simulink model "motor3"  (R2021a)
settings: Solver=VariableStepAuto  StartTime=0.0  StopTime=10.0  RelTol=1e-3
libraries: nesl_utility x12, ee_lib x10, fl_lib x7, pid_lib x3, eeTransforms x2, embmathops x2, eePwmGeneratorTwoLevel x1
settings Model: Creator=Sujit  LastModifiedBy=Sujit

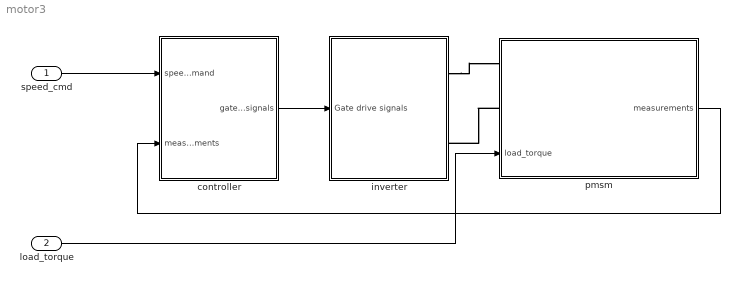
== system motor3 ==
  speed_cmd : Inport
  load_torque : Inport  Port=2
  controller : Subsystem
  inverter : Subsystem
  pmsm : Subsystem
      settings: PortSchema="{\"entries\":[{\"content\":{\"sides\":[{\"content\":{\"connectorIds\":[\"LConn1\",\"LConn2\",\"In1\"]},\"type\":\"ConnectorPlacement.EquallySpacedRectSide\",\"uuid\":\"9aa95156-5b90-445e-ac58-1a81c189d6db\"},{\"content\":{\"connectorIds\":[\"Out1\"],\"side\":\"RIGHT\"},\"type\":\"ConnectorPlacement.EquallySpacedRectSide\",\"uuid\":\"e0f82fa8-5145-4e03-9494-9a86df107329\"},{\"content\":{\"connectorIds\":[],\"side\":\"TOP\"},\"type\":\"ConnectorPlacement.EquallySpacedRectSide\",\"uuid\":\"ed322135-5092-4528-967b-f1137f8969df\"}]},\"type\":\"ConnectorPlacement.EquallySpacedConnector\",\"uuid\":\"a6e6cb3b-bfcb-454a-ab1c-5c06ba05c769\"}],\"packageUris\":[\"http://schema.mathworks.com/mf0/Connector/R2020b\"],\"version\":\"1.0\"}"
  wires:
  load_torque/1 -> pmsm/1(load_torque)
  pmsm/1(measurements) -> controller/2(measurements)
  speed_cmd/1 -> controller/1(speed_command)
  controller/1(gate_signals) -> inverter/1(Gate drive signals)
  connections:
  inverter/RConn1 -- pmsm/LConn1
  pmsm/LConn2 -- inverter/RConn2

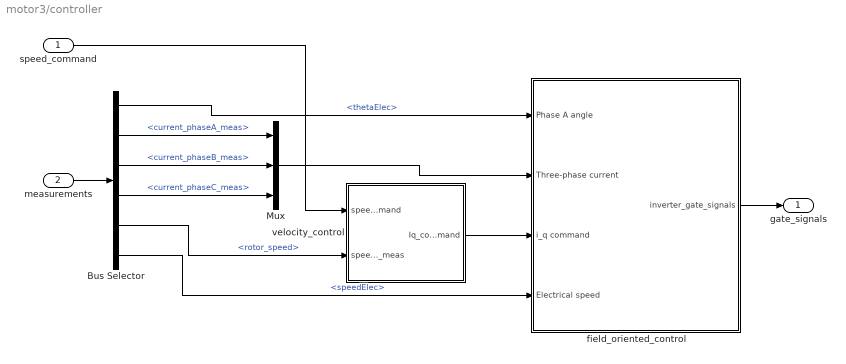
== system motor3/controller ==
  speed_command : Inport
  measurements : Inport  Port=2
  Bus Selector : BusSelector  OutputSignals=thetaElec,current_phaseA_meas,current_phaseB_meas,current_phaseC_meas,rotor_speed,speedElec
  Mux : Mux  Inputs=3
  field_oriented_control : Subsystem
  velocity_control : Subsystem
  gate_signals : Outport
  wires:
  velocity_control/1(Iq_command) -> field_oriented_control/3(i_q command)
  speed_command/1 -> velocity_control/1(speed_command)
  measurements/1 -> Bus Selector/1
  Bus Selector/5 -> velocity_control/2(speed_meas)  "<rotor_speed>"
  Bus Selector/2 -> Mux/1  "<current_phaseA_meas>"
  Bus Selector/3 -> Mux/2  "<current_phaseB_meas>"
  Bus Selector/4 -> Mux/3  "<current_phaseC_meas>"
  Mux/1 -> field_oriented_control/2(Three-phase current)
  field_oriented_control/1(inverter_gate_signals) -> gate_signals/1
  Bus Selector/1 -> field_oriented_control/1(Phase A angle)  "<thetaElec>"
  Bus Selector/6 -> field_oriented_control/4(Electrical speed)  "<speedElec>"

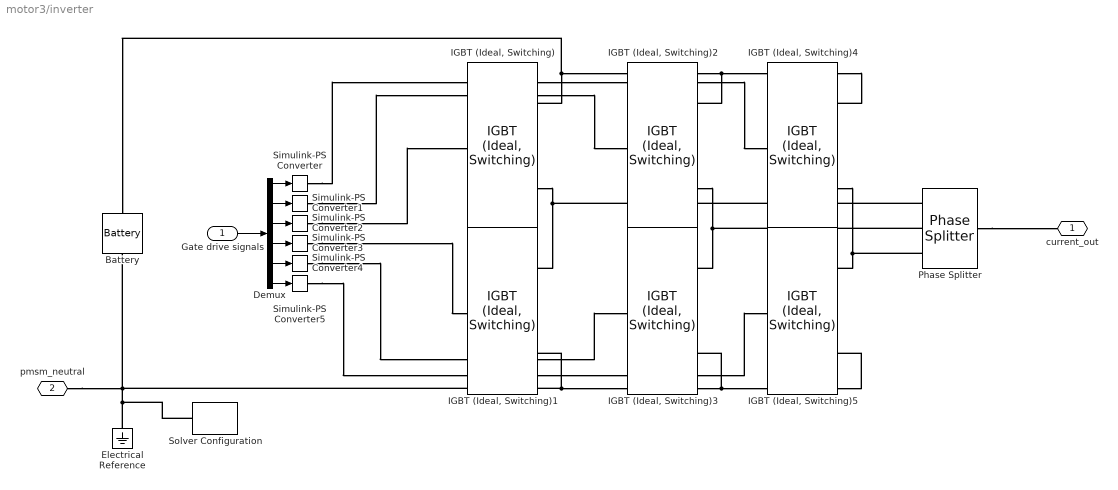
== system motor3/inverter ==
  Gate drive signals : Inport
  Battery : ee_lib/Sources/Battery  Vnom=400 V  prm_dir=1  R1_dis=2 Ohm  R1_ch=2 Ohm  R1=2 Ohm  prm_AH=1  AH=50 hr*A  V1=11.5 V  AH1=25 hr*A  prm_R2=1  R2=2000 Ohm  prm_dyn=1  Rp1=0.005 Ohm  tau1=30 s  Rp2=0.005 Ohm  tau2=30 s  Rp3=0.005 Ohm  tau3=30 s  Rp4=0.005 Ohm  tau4=30 s  Rp5=0.005 Ohm  tau5=30 s  prm_fade=1  N_fade=100  AH_fade=45 hr*A  R1_fade=2.02 Ohm  R1_ch_fade=2.02 Ohm  V1_fade=10.35 V  prm_age=1  prm_age_OCV=1  OCV_age=0.9  SOC_age=60  Tmeas_age=298.15 K  delta_time_age_vec=[0] d  temperature_age_vec=[273] K  OCV_scaling_age=2.2134e6  OCV_offset_age=1.632e6  temp_exp_age=0.515833569 V  t_exp_age=0.75  i_specify=off  i_priority=None  i=0 A  i_nominal_specify=off  i_nominal_unit=A  i_nominal_value=1  v_specify=off  v_priority=None  v=0 V  v_nominal_specify=off  v_nominal_unit=V  v_nominal_value=1  charge_specify=off  charge_priority=High  charge=50 hr*A  charge_nominal_specify=off  charge_nominal_unit=hr*A  charge_nominal_value=1  num_cycles_specify=off  num_cycles_priority=High  num_cycles=0  num_cycles_nominal_specify=off  num_cycles_nominal_unit=1  num_cycles_nominal_value=1  thermal_mass=30000 J/K  Tmeas=298.15 K  Vnom_T2=12 V  R1_T2=2.2 Ohm  R1_T2_dis=2.2 Ohm  R1_T2_ch=2.2 Ohm  V1_T2=11.4 V  R2_T2=2200 Ohm  Rp1_T2=0.005 Ohm  tau1_T2=30 s  Rp2_T2=0.005 Ohm  tau2_T2=30 s  Rp3_T2=0.005 Ohm  tau3_T2=30 s  Rp4_T2=0.005 Ohm  tau4_T2=30 s  Rp5_T2=0.005 Ohm  tau5_T2=30 s  Tmeas2=273.15 K  temperature_specify=off  temperature_priority=High  temperature=298.15 K  temperature_nominal_specify=off  temperature_nominal_unit=K  temperature_nominal_value=1
  Demux : Demux  Outputs=6
  Electrical Reference : fl_lib/Electrical/Electrical Elements/Electrical Reference
  IGBT (Ideal, Switching){,1..5} (6 alike) : ee_lib/Semiconductors & Converters/IGBT (Ideal, Switching)  Vf=0.8 V  Ron=0.021 Ohm  Goff=0.12195 1/Ohm  Vth=5.8 V  diode_param=ee.enum.converters.protectiondiode.chargedynamics  diode_Vf=2.22 V  diode_Ron=0.0184 Ohm  diode_Goff=1 1/Ohm  diode_C=50e-9 F  diode_iRM=-35 A  diode_iF=50 A  diode_idot=-1380 A/us  diode_trr_param=ee.enum.converters.diodetrr.Qrr  diode_trr_factor=3  diode_trr=15 us  diode_Qrr=8.7 uC  thermal_loss_option=ee.enum.converters.thermalLossOption.constantvalues  Von_data=[0, .1, .6, .8, 1, 1.3, 1.6, 2, 2.4; 0, .1, .7, 1, 1.2, 1.5, 1.9, 2.4, 2.8] V  Eon_data=[0, .0024, .024, .12, .2, .48, 1.04, 2.16, 3.24; 0, .003, .03, .15, .25, .6, 1.3, 2.7, 4.05] * 1e-3 J  Eoff_data=[0, .0007, .0066, .033, .066, .17, .33, .83, 1.5; 0, .001, .01, .05, .1, .25, .5, 1.2, 2.2] * 1e-3 J  Tj=[298.15, 398.15] K  Iout_data=[0, .1, 1, 5, 10, 20, 40, 70, 100] A  Eon_scalar=5.5e-3 J  Eoff_scalar=4.5e-3 J  Voff=600 V  Iout_scalar=50 A  diodeModelType=ee.enum.converters.diodeModelType.pwl  diode_IfMat=[.07, .12, .19, 1.75, 4.24, 7.32, 11.2; .16, .3, .72, 2.14, 4.02, 6.35, 9.12] A  diode_TjVec=[25, 125] degC  diode_VfVec=[.5, .7, .9, 1.3, 1.7, 2.1, 2.5] V  thermal_network_parameterization=ee.enum.thermalNetworkTopology.cauer  Rth=[.53, .5] K/W  Rth_Foster=[.08, .14, .22, .16] K/W  thermal_mass_parameterization=ee.enum.thermalNetwork.timeconstant  thermal_mass=[.01, .5] J/K  thermal_mass_Foster=[.001, .005, .05, .5] J/K  thermal_time_constant=[.001, .2] s  thermal_time_constant_Foster=[7e-05, .0007, .01, .08] s  thermal_mass_initial_temperatures=[25, 25] degC  junction_thermal_mass=0.01 J/K  vT_specify=off  vT_priority=None  vT=0 V  vT_nominal_specify=off  vT_nominal_unit=V  vT_nominal_value=1  Qj_specify=off  Qj_priority=None  Qj=0 W  Qj_nominal_specify=off  Qj_nominal_unit=W  Qj_nominal_value=1  junction_temperature_specify=on  junction_temperature_priority=None  junction_temperature=25 degC  junction_temperature_nominal_specify=off  junction_temperature_nominal_unit=degC  junction_temperature_nominal_value=1
  Phase Splitter : ee_lib/Connectors & References/Phase Splitter
      settings: SourceProductBaseCode=PS
  Simulink-PS Converter{,1..5} (6 alike) : nesl_utility/Simulink-PS Converter  PhysicalDomain=network_engine_domain  SubClassName=ps_input  LeftPortType=input  RightPortType=output  PseudoPeriodic=off  Frequencies=[]  NoiseDistribution=none  NoiseParameters=[]  Unit=1  AffineConversion=off  FilteringAndDerivatives=provide  SimscapeFilterOrder=1  InputFilterTimeConstant=0.001  UdotUserProvided=0
      settings: SourceProductBaseCode=PW,SS
  Solver Configuration : nesl_utility/Solver Configuration  PhysicalDomain=network_engine_domain  SubClassName=solver  LeftPortType=input  RightPortType=generic  Tones=[]  Harmonics=[]  SimulateNoise=off  Profile=off  UseLocalSampling=off  EnableSwitchedLinearOptims=on  FrequencyDomain=off  UseCCode=off  RelTol=0.001  AbsTol=1e-06  MinStep=1e-09  ToWorkspace=off  RevertToSquareIcSolve=off  NumHomotopyIterations=100  PhasorMode=off  PhasorModeNumHarmonics=1  DoDC=off  ResidualTolerance=1e-09  UseLocalSolver=off  LocalSolverChoice=NE_BACKWARD_EULER_ADVANCER  LocalSolverSampleTime=0.001  DoFixedCost=off  MaxNonlinIter=3  MaxModeIter=2  ComputeImpulses=off  ImpulseIterations=2  LinearAlgebra=auto  EquationFormulation=NE_TIME_EF  DelaysMemoryBudget=1024  AutomaticFiltering=on  FilteringTimeConstant=0.001  PartitionStorageMethod=AS_NEEDED  PartitionMemoryBudget=1024  PartitionMethod=ROBUST
      settings: SourceProductBaseCode=PW,SS
  current_out : PMIOPort  Side=Right
  pmsm_neutral : PMIOPort  Port=2  Side=Right
  wires:
  Demux/1 -> Simulink-PS Converter/1
  Demux/2 -> Simulink-PS Converter1/1
  Demux/6 -> Simulink-PS Converter5/1
  Demux/3 -> Simulink-PS Converter2/1
  Demux/4 -> Simulink-PS Converter3/1
  Demux/5 -> Simulink-PS Converter4/1
  Gate drive signals/1 -> Demux/1
  connections:
  "IGBT (Ideal, Switching)2"/RConn2 -- Phase Splitter/RConn2 -- "IGBT (Ideal, Switching)3"/RConn1
  Battery/LConn1 -- "IGBT (Ideal, Switching)"/RConn1 -- "IGBT (Ideal, Switching)4"/RConn1 -- "IGBT (Ideal, Switching)2"/RConn1
  Solver Configuration/RConn1 -- Electrical Reference/LConn1 -- pmsm_neutral/RConn1 -- Battery/RConn1 -- "IGBT (Ideal, Switching)1"/RConn2 -- "IGBT (Ideal, Switching)5"/RConn2 -- "IGBT (Ideal, Switching)3"/RConn2
  "IGBT (Ideal, Switching)"/RConn2 -- Phase Splitter/RConn1 -- "IGBT (Ideal, Switching)1"/RConn1
  "IGBT (Ideal, Switching)4"/RConn2 -- Phase Splitter/RConn3 -- "IGBT (Ideal, Switching)5"/RConn1
  Simulink-PS Converter/RConn1 -- "IGBT (Ideal, Switching)4"/LConn1
  Simulink-PS Converter1/RConn1 -- "IGBT (Ideal, Switching)2"/LConn1
  Simulink-PS Converter2/RConn1 -- "IGBT (Ideal, Switching)"/LConn1
  Simulink-PS Converter3/RConn1 -- "IGBT (Ideal, Switching)1"/LConn1
  Simulink-PS Converter4/RConn1 -- "IGBT (Ideal, Switching)3"/LConn1
  Simulink-PS Converter5/RConn1 -- "IGBT (Ideal, Switching)5"/LConn1
  Phase Splitter/LConn1 -- current_out/RConn1

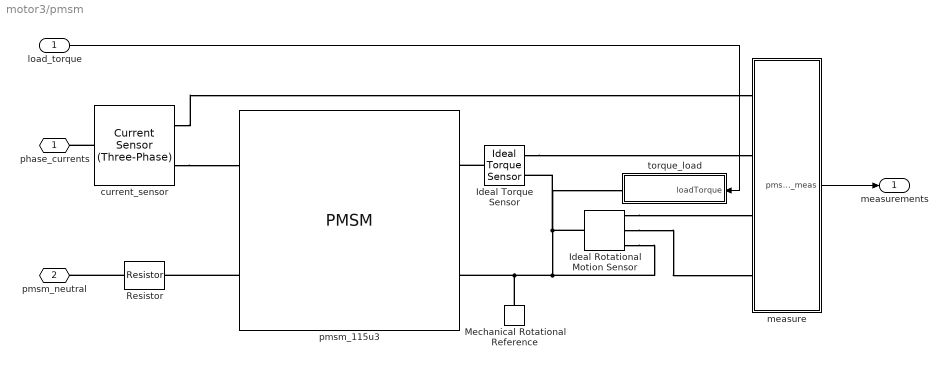
== system motor3/pmsm ==
  load_torque : Inport
  Ideal Rotational Motion Sensor : fl_lib/Mechanical/Mechanical Sensors/Ideal Rotational Motion Sensor  wrap_angle=simscape.enum.onoff.off  offset=0 rad
  Ideal Torque Sensor : fl_lib/Mechanical/Mechanical Sensors/Ideal Torque Sensor
  Mechanical Rotational Reference : fl_lib/Mechanical/Rotational Elements/Mechanical Rotational Reference
  Resistor : fl_lib/Electrical/Electrical Elements/Resistor  R=1000 Ohm  i_specify=off  i_priority=None  i=0 A  i_nominal_specify=off  i_nominal_unit=A  i_nominal_value=1  v_specify=off  v_priority=None  v=0 V  v_nominal_specify=off  v_nominal_unit=V  v_nominal_value=1
  current_sensor : ee_lib/Sensors & Transducers/Current Sensor (Three-Phase)
  measure : Subsystem
  pmsm_115u3 : ee_lib/Electromechanical/Permanent Magnet/PMSM  winding_type=ee.enum.statorconnection.wye  machine_param=ee.enum.pmsm.parameterization.constant  nPolePairs=6  pmflux_param=ee.enum.pmflux.fluxlinkage  pm_flux_linkage=0.03 Wb  torque_constant=0.18 N*m/A  back_emf_constant=0.18 V/(rad/s)  stator_param=ee.enum.statorparam.LdLqL0  Ld=0.00019 H  Lq=0.00025 H  idVec=[-200, 0, 200] A  iqVec=[-200, 0, 200] A  LdMatrix=0.0002 * ones(3, 3) H  LqMatrix=0.0002 * ones(3, 3) H  PmMatrix=0.1 * ones(3, 3) Wb  ktMatrix=0.18 * ones(3, 3) N*m/A  keMatrix=0.18 * ones(3, 3) V/(rad/s)  L0=0.00016 H  Ls=0.0002 H  Lm=-0.00002 H  Ms=0.00002 H  Rs=0.013 Ohm  zero_sequence=ee.enum.park.zerosequence.include  J=0.01 kg*m^2  lam=0 N*m/(rad/s)  axes_param=ee.enum.rotorangle.daxis  i_d_specify=off  i_d_priority=None  i_d=0 A  i_d_nominal_specify=off  i_d_nominal_unit=A  i_d_nominal_value=1  i_q_specify=off  i_q_priority=None  i_q=0 A  i_q_nominal_specify=off  i_q_nominal_unit=A  i_q_nominal_value=1  torque_specify=off  torque_priority=None  torque=0 N*m  torque_nominal_specify=off  torque_nominal_unit=N*m  torque_nominal_value=1  angular_velocity_specify=off  angular_velocity_priority=High  angular_velocity=0 rpm  angular_velocity_nominal_specify=off  angular_velocity_nominal_unit=rpm  angular_velocity_nominal_value=1  angular_position_specify=off  angular_position_priority=High  angular_position=0 deg  angular_position_nominal_specify=off  angular_position_nominal_unit=deg  angular_position_nominal_value=1  loss_param=ee.enum.ironloss.none  losses_oc=[0, 0, 0] W  losses_sc=[0, 0, 0] W  f_losses=60 Hz  Isc_losses=95 A  Tmeas=298.15 K  alpha=3.93e-3 1/K  alpha_flux=-0.001 1/K  stator_thermal_mass=100 J/K  rotor_thermal_mass=200 J/K  Rm_percent_rotor=90  Rd_percent_rotor=30  temperatureA_specify=off  temperatureA_priority=High  temperatureA=25 degC  temperatureA_nominal_specify=off  temperatureA_nominal_unit=degC  temperatureA_nominal_value=1  temperatureB_specify=off  temperatureB_priority=High  temperatureB=25 degC  temperatureB_nominal_specify=off  temperatureB_nominal_unit=degC  temperatureB_nominal_value=1  temperatureC_specify=off  temperatureC_priority=High  temperatureC=25 degC  temperatureC_nominal_specify=off  temperatureC_nominal_unit=degC  temperatureC_nominal_value=1  temperatureR_specify=off  temperatureR_priority=High  temperatureR=25 degC  temperatureR_nominal_specify=off  temperatureR_nominal_unit=degC  temperatureR_nominal_value=1
      settings: InternalSimscapePortConfiguration="{\"Bottom\":[],\"Left\":[{\"id\":\"N\",\"label\":\"~\",\"type\":\"foundation.electrical.three_phase\"},{\"id\":\"n\",\"label\":\"n\",\"type\":\"foundation.electrical.electrical\"}],\"Right\":[{\"id\":\"R\",\"label\":\"R\",\"type\":\"foundation.mechanical.rotational.rotational\"},{\"id\":\"C\",\"label\":\"C\",\"type\":\"foundation.mechanical.rotational.rotational\"}],\"Top\":[]}"
  torque_load : Subsystem
      settings: PortSchema="{\"entries\":[{\"content\":{\"sides\":[{\"content\":{\"connectorIds\":[\"LConn1\"]},\"type\":\"ConnectorPlacement.EquallySpacedRectSide\",\"uuid\":\"e4784f29-d93f-4577-9aa6-c4ef50a9b071\"},{\"content\":{\"connectorIds\":[\"In1\"],\"side\":\"RIGHT\"},\"type\":\"ConnectorPlacement.EquallySpacedRectSide\",\"uuid\":\"89d2c505-8cad-412e-9073-9a6566c773aa\"},{\"content\":{\"connectorIds\":[],\"side\":\"TOP\"},\"type\":\"ConnectorPlacement.EquallySpacedRectSide\",\"uuid\":\"f7c01527-04e7-4eb1-8d66-c3862d981b69\"}]},\"type\":\"ConnectorPlacement.EquallySpacedConnector\",\"uuid\":\"d5a2cd28-8ac4-473c-b7d1-ef94d8c3a580\"}],\"packageUris\":[\"http://schema.mathworks.com/mf0/Connector/R2020b\"],\"version\":\"1.0\"}"
  phase_currents : PMIOPort  Side=Left
  pmsm_neutral : PMIOPort  Port=2  Side=Left
  measurements : Outport
  wires:
  measure/1(pmsm_meas) -> measurements/1
  load_torque/1 -> torque_load/1(loadTorque)
  connections:
  Ideal Rotational Motion Sensor/RConn3 -- measure/LConn3
  Ideal Torque Sensor/RConn2 -- measure/LConn2
  Ideal Rotational Motion Sensor/LConn1 -- Ideal Torque Sensor/RConn1 -- torque_load/LConn1 -- Mechanical Rotational Reference/LConn1 -- pmsm_115u3/RConn2 -- Ideal Rotational Motion Sensor/RConn1
  current_sensor/RConn2 -- pmsm_115u3/LConn1
  current_sensor/RConn1 -- measure/LConn1
  Ideal Rotational Motion Sensor/RConn2 -- measure/LConn4
  Ideal Torque Sensor/LConn1 -- pmsm_115u3/RConn1
  Resistor/LConn1 -- pmsm_neutral/RConn1
  current_sensor/LConn1 -- phase_currents/RConn1
  pmsm_115u3/LConn2 -- Resistor/RConn1

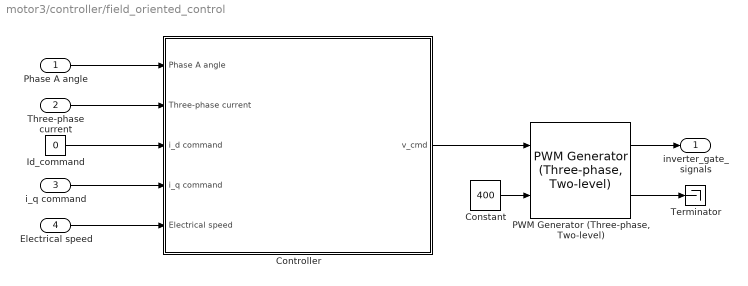
== system motor3/controller/field_oriented_control ==
  Phase A angle : Inport
  Three-phase current : Inport  Port=2
  i_q command : Inport  Port=3
  Electrical speed : Inport  Port=4
  Constant : Constant  Value=400
  Controller : Subsystem
  Id_command : Constant  Value=0
  "PWM Generator (Three-phase, Two-level)" : eePwmGeneratorTwoLevel/PWM Generator (Three-phase, Two-level)  PWMMode=Continuous PWM (CPWM)  CPWMMode=SPWM: sinusoidal PWM  DPWMMode=60 DPWM: 60 degree discontinuous PWM  fsw=1e3  Ts=5e-5
      settings: SourceProductBaseCode=PS
  Terminator : Terminator
  inverter_gate_signals : Outport
  wires:
  Phase A angle/1 -> Controller/1(Phase A angle)
  Three-phase current/1 -> Controller/2(Three-phase current)
  Id_command/1 -> Controller/3(i_d command)
  i_q command/1 -> Controller/4(i_q command)
  Electrical speed/1 -> Controller/5(Electrical speed)
  "PWM Generator (Three-phase, Two-level)"/1 -> inverter_gate_signals/1
  Constant/1 -> "PWM Generator (Three-phase, Two-level)"/2
  Controller/1(v_cmd) -> "PWM Generator (Three-phase, Two-level)"/1
  "PWM Generator (Three-phase, Two-level)"/2 -> Terminator/1

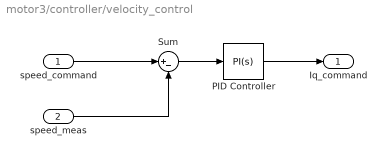
== system motor3/controller/velocity_control ==
  speed_command : Inport
  speed_meas : Inport  Port=2
  PID Controller : pid_lib/PID Controller  Controller=PI  Form=Parallel  TimeDomain=Continuous-time  UseExternalTs=off  SampleTime=-1  IntegratorMethod=Forward Euler  FilterMethod=Forward Euler  ControllerParametersSource=internal  P=1  I=1  D=0  UseFilter=on  N=100  TunerSelectOption=Transfer Function Based (PID Tuner App)  InitialConditionSource=internal  InitialConditionForIntegrator=0  InitialConditionForFilter=0  DifferentiatorICPrevScaledInput=0  ExternalReset=none  TrackingMode=off  Kt=1  LimitOutput=off  SatLimitsSource=internal  UpperSaturationLimit=inf  LowerSaturationLimit=-inf  LinearizeAsGain=on  AntiWindupMode=none  Kb=1  POutMin=[]  POutMax=[]  IOutMin=[]  IOutMax=[]  DOutMin=[]  DOutMax=[]  NOutMin=[]  NOutMax=[]  SumOutMin=[]  SumOutMax=[]  SaturationOutMin=[]  SaturationOutMax=[]  PParamMin=[]  PParamMax=[]  IParamMin=[]  IParamMax=[]  DParamMin=[]  DParamMax=[]  NParamMin=[]  NParamMax=[]  KbParamMin=[]  KbParamMax=[]  KtParamMin=[]  KtParamMax=[]  KbOutMin=[]  KbOutMax=[]  KtOutMin=[]  KtOutMax=[]  IntegratorOutMin=[]  IntegratorOutMax=[]  FilterOutMin=[]  FilterOutMax=[]  SumI1OutMin=[]  SumI1OutMax=[]  SumI2OutMin=[]  SumI2OutMax=[]  SumI3OutMin=[]  SumI3OutMax=[]  SumI4OutMin=[]  SumI4OutMax=[]  SumDOutMin=[]  SumDOutMax=[]  DifferentiatorOutMin=[]  DifferentiatorOutMax=[]  FilterDiffOutCoefMin=[]  FilterDiffOutCoefMax=[]  ReciprocalOutMin=[]  ReciprocalOutMax=[]  SumDenOutMin=[]  SumDenOutMax=[]  SumNumOutMin=[]  SumNumOutMax=[]  DivideOutMin=[]  DivideOutMax=[]  UdiffTsProdOutMin=[]  UdiffTsProdOutMax=[]  NTsProdOutMin=[]  NTsProdOutMax=[]  UintegralTsProdOutMin=[]  UintegralTsProdOutMax=[]  UngainTsProdOutMin=[]  UngainTsProdOutMax=[]  IntegratorContinuousStateAttributes=''  IntegratorStateMustResolveToSignalObject=off  IntegratorRTWStateStorageClass=Auto  FilterContinuousStateAttributes=''  FilterStateMustResolveToSignalObject=off  FilterRTWStateStorageClass=Auto  ParallelPVariant=InternalParameters  IdealPVariant=Disabled  IVariant=InternalParameters  DVariant=Disabled  IntegratorVariant=Continuous  SatVariant=Disabled  AWVariant=Passthrough  PCopyVariant=Disabled  TRVariant=Disabled  FdbkBlocksVariant=Forward  IdealPFdbkVariant=Disabled  SatFdbkVariant=Disabled  DerivativeFilterVariant=Disabled  NVariant=Disabled  NCopyVariant=Disabled_SignalSpec  FilterICVariant=Disabled  IntegratorICVariant=InternalICs  ExternalResetVariant=Disabled  TRSumVariant=Passthrough  SumFdbkVariant=Disabled  SumVariant=Sum_PI  TsampFilterVariant=InternalTs  TsampNgainVariant=Passthrough  TsampIntegralVariant=Passthrough  ExternalSaturationOutDataTypeStr=Inherit: Same as second input
  Sum : Sum  Inputs=|+-
  Iq_command : Outport
  wires:
  speed_meas/1 -> Sum/2
  speed_command/1 -> Sum/1
  Sum/1 -> PID Controller/1
  PID Controller/1 -> Iq_command/1

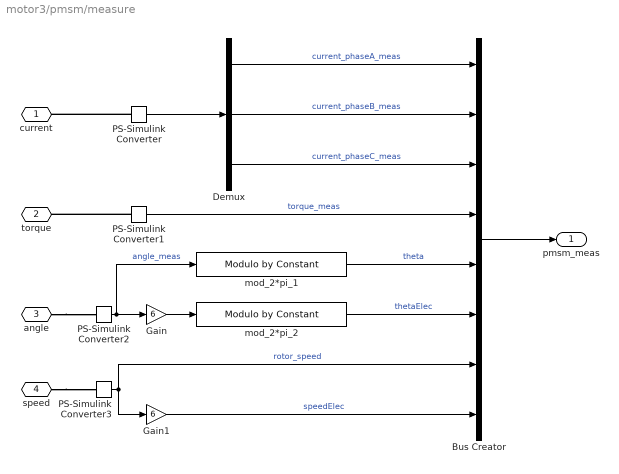
== system motor3/pmsm/measure ==
  Bus Creator : BusCreator  Inputs=8
  Demux : Demux  Outputs=3
  Gain : Gain  Gain=6
  Gain1 : Gain  Gain=6
  PS-Simulink Converter{,1..3} (4 alike) : nesl_utility/PS-Simulink Converter  PhysicalDomain=network_engine_domain  SubClassName=ps_output  LeftPortType=input  RightPortType=output  PseudoPeriodic=off  Frequencies=[]  Unit=inherit  AffineConversion=off
      settings: SourceProductBaseCode=PW,SS
  mod_2*pi_1 : embmathops/Modulo by Constant  Denominator=2*pi  SimulateUsing=Code generation
      settings: SourceProductBaseCode=SL
  mod_2*pi_2 : embmathops/Modulo by Constant  Denominator=2*pi  SimulateUsing=Code generation
      settings: SourceProductBaseCode=SL
  current : PMIOPort  Side=Left
  torque : PMIOPort  Port=2  Side=Left
  angle : PMIOPort  Port=3  Side=Left
  speed : PMIOPort  Port=4  Side=Left
  pmsm_meas : Outport
  wires:
  PS-Simulink Converter/1 -> Demux/1
  PS-Simulink Converter1/1 -> Bus Creator/4  "torque_meas"
  PS-Simulink Converter3/1 -> Gain1/1, Bus Creator/7  "rotor_speed"
  PS-Simulink Converter2/1 -> Gain/1, mod_2*pi_1/1  "angle_meas"
  Demux/1 -> Bus Creator/1  "current_phaseA_meas"
  Demux/2 -> Bus Creator/2  "current_phaseB_meas"
  Demux/3 -> Bus Creator/3  "current_phaseC_meas"
  Bus Creator/1 -> pmsm_meas/1
  mod_2*pi_1/1 -> Bus Creator/5  "theta"
  Gain/1 -> mod_2*pi_2/1
  mod_2*pi_2/1 -> Bus Creator/6  "thetaElec"
  Gain1/1 -> Bus Creator/8  "speedElec"
  connections:
  PS-Simulink Converter/LConn1 -- current/RConn1
  PS-Simulink Converter1/LConn1 -- torque/RConn1
  angle/RConn1 -- PS-Simulink Converter2/LConn1
  speed/RConn1 -- PS-Simulink Converter3/LConn1

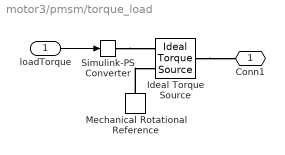
== system motor3/pmsm/torque_load ==
  loadTorque : Inport
  Ideal Torque Source : fl_lib/Mechanical/Mechanical Sources/Ideal Torque Source
  Mechanical Rotational Reference : fl_lib/Mechanical/Rotational Elements/Mechanical Rotational Reference
  Simulink-PS Converter : nesl_utility/Simulink-PS Converter  PhysicalDomain=network_engine_domain  SubClassName=ps_input  LeftPortType=input  RightPortType=output  PseudoPeriodic=off  Frequencies=[]  NoiseDistribution=none  NoiseParameters=[]  Unit=1  AffineConversion=off  FilteringAndDerivatives=provide  SimscapeFilterOrder=1  InputFilterTimeConstant=0.001  UdotUserProvided=0
      settings: SourceProductBaseCode=PW,SS
  Conn1 : PMIOPort  Side=Left
  wires:
  loadTorque/1 -> Simulink-PS Converter/1
  connections:
  Mechanical Rotational Reference/LConn1 -- Ideal Torque Source/RConn2
  Ideal Torque Source/LConn1 -- Conn1/RConn1
  Simulink-PS Converter/RConn1 -- Ideal Torque Source/RConn1

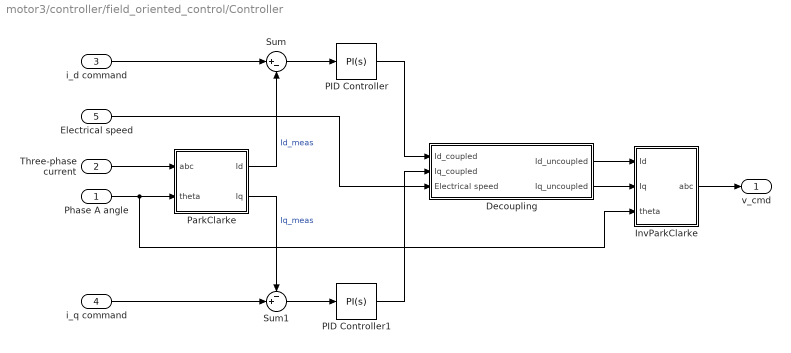
== system motor3/controller/field_oriented_control/Controller ==
  Phase A angle : Inport
  Three-phase current : Inport  Port=2
  i_d command : Inport  Port=3
  i_q command : Inport  Port=4
  Electrical speed : Inport  Port=5
  Decoupling : Subsystem
  InvParkClarke : Subsystem
  PID Controller : pid_lib/PID Controller  Controller=PI  Form=Parallel  TimeDomain=Continuous-time  UseExternalTs=off  SampleTime=-1  IntegratorMethod=Forward Euler  FilterMethod=Forward Euler  ControllerParametersSource=internal  P=1  I=1  D=0  UseFilter=on  N=100  TunerSelectOption=Transfer Function Based (PID Tuner App)  InitialConditionSource=internal  InitialConditionForIntegrator=0  InitialConditionForFilter=0  DifferentiatorICPrevScaledInput=0  ExternalReset=none  TrackingMode=off  Kt=1  LimitOutput=off  SatLimitsSource=internal  UpperSaturationLimit=inf  LowerSaturationLimit=-inf  LinearizeAsGain=on  AntiWindupMode=none  Kb=1  POutMin=[]  POutMax=[]  IOutMin=[]  IOutMax=[]  DOutMin=[]  DOutMax=[]  NOutMin=[]  NOutMax=[]  SumOutMin=[]  SumOutMax=[]  SaturationOutMin=[]  SaturationOutMax=[]  PParamMin=[]  PParamMax=[]  IParamMin=[]  IParamMax=[]  DParamMin=[]  DParamMax=[]  NParamMin=[]  NParamMax=[]  KbParamMin=[]  KbParamMax=[]  KtParamMin=[]  KtParamMax=[]  KbOutMin=[]  KbOutMax=[]  KtOutMin=[]  KtOutMax=[]  IntegratorOutMin=[]  IntegratorOutMax=[]  FilterOutMin=[]  FilterOutMax=[]  SumI1OutMin=[]  SumI1OutMax=[]  SumI2OutMin=[]  SumI2OutMax=[]  SumI3OutMin=[]  SumI3OutMax=[]  SumI4OutMin=[]  SumI4OutMax=[]  SumDOutMin=[]  SumDOutMax=[]  DifferentiatorOutMin=[]  DifferentiatorOutMax=[]  FilterDiffOutCoefMin=[]  FilterDiffOutCoefMax=[]  ReciprocalOutMin=[]  ReciprocalOutMax=[]  SumDenOutMin=[]  SumDenOutMax=[]  SumNumOutMin=[]  SumNumOutMax=[]  DivideOutMin=[]  DivideOutMax=[]  UdiffTsProdOutMin=[]  UdiffTsProdOutMax=[]  NTsProdOutMin=[]  NTsProdOutMax=[]  UintegralTsProdOutMin=[]  UintegralTsProdOutMax=[]  UngainTsProdOutMin=[]  UngainTsProdOutMax=[]  IntegratorContinuousStateAttributes=''  IntegratorStateMustResolveToSignalObject=off  IntegratorRTWStateStorageClass=Auto  FilterContinuousStateAttributes=''  FilterStateMustResolveToSignalObject=off  FilterRTWStateStorageClass=Auto  ParallelPVariant=InternalParameters  IdealPVariant=Disabled  IVariant=InternalParameters  DVariant=Disabled  IntegratorVariant=Continuous  SatVariant=Disabled  AWVariant=Passthrough  PCopyVariant=Disabled  TRVariant=Disabled  FdbkBlocksVariant=Forward  IdealPFdbkVariant=Disabled  SatFdbkVariant=Disabled  DerivativeFilterVariant=Disabled  NVariant=Disabled  NCopyVariant=Disabled_SignalSpec  FilterICVariant=Disabled  IntegratorICVariant=InternalICs  ExternalResetVariant=Disabled  TRSumVariant=Passthrough  SumFdbkVariant=Disabled  SumVariant=Sum_PI  TsampFilterVariant=InternalTs  TsampNgainVariant=Passthrough  TsampIntegralVariant=Passthrough  ExternalSaturationOutDataTypeStr=Inherit: Same as second input
  PID Controller1 : pid_lib/PID Controller  Controller=PI  Form=Parallel  TimeDomain=Continuous-time  UseExternalTs=off  SampleTime=-1  IntegratorMethod=Forward Euler  FilterMethod=Forward Euler  ControllerParametersSource=internal  P=1  I=1  D=0  UseFilter=on  N=100  TunerSelectOption=Transfer Function Based (PID Tuner App)  InitialConditionSource=internal  InitialConditionForIntegrator=0  InitialConditionForFilter=0  DifferentiatorICPrevScaledInput=0  ExternalReset=none  TrackingMode=off  Kt=1  LimitOutput=off  SatLimitsSource=internal  UpperSaturationLimit=inf  LowerSaturationLimit=-inf  LinearizeAsGain=on  AntiWindupMode=none  Kb=1  POutMin=[]  POutMax=[]  IOutMin=[]  IOutMax=[]  DOutMin=[]  DOutMax=[]  NOutMin=[]  NOutMax=[]  SumOutMin=[]  SumOutMax=[]  SaturationOutMin=[]  SaturationOutMax=[]  PParamMin=[]  PParamMax=[]  IParamMin=[]  IParamMax=[]  DParamMin=[]  DParamMax=[]  NParamMin=[]  NParamMax=[]  KbParamMin=[]  KbParamMax=[]  KtParamMin=[]  KtParamMax=[]  KbOutMin=[]  KbOutMax=[]  KtOutMin=[]  KtOutMax=[]  IntegratorOutMin=[]  IntegratorOutMax=[]  FilterOutMin=[]  FilterOutMax=[]  SumI1OutMin=[]  SumI1OutMax=[]  SumI2OutMin=[]  SumI2OutMax=[]  SumI3OutMin=[]  SumI3OutMax=[]  SumI4OutMin=[]  SumI4OutMax=[]  SumDOutMin=[]  SumDOutMax=[]  DifferentiatorOutMin=[]  DifferentiatorOutMax=[]  FilterDiffOutCoefMin=[]  FilterDiffOutCoefMax=[]  ReciprocalOutMin=[]  ReciprocalOutMax=[]  SumDenOutMin=[]  SumDenOutMax=[]  SumNumOutMin=[]  SumNumOutMax=[]  DivideOutMin=[]  DivideOutMax=[]  UdiffTsProdOutMin=[]  UdiffTsProdOutMax=[]  NTsProdOutMin=[]  NTsProdOutMax=[]  UintegralTsProdOutMin=[]  UintegralTsProdOutMax=[]  UngainTsProdOutMin=[]  UngainTsProdOutMax=[]  IntegratorContinuousStateAttributes=''  IntegratorStateMustResolveToSignalObject=off  IntegratorRTWStateStorageClass=Auto  FilterContinuousStateAttributes=''  FilterStateMustResolveToSignalObject=off  FilterRTWStateStorageClass=Auto  ParallelPVariant=InternalParameters  IdealPVariant=Disabled  IVariant=InternalParameters  DVariant=Disabled  IntegratorVariant=Continuous  SatVariant=Disabled  AWVariant=Passthrough  PCopyVariant=Disabled  TRVariant=Disabled  FdbkBlocksVariant=Forward  IdealPFdbkVariant=Disabled  SatFdbkVariant=Disabled  DerivativeFilterVariant=Disabled  NVariant=Disabled  NCopyVariant=Disabled_SignalSpec  FilterICVariant=Disabled  IntegratorICVariant=InternalICs  ExternalResetVariant=Disabled  TRSumVariant=Passthrough  SumFdbkVariant=Disabled  SumVariant=Sum_PI  TsampFilterVariant=InternalTs  TsampNgainVariant=Passthrough  TsampIntegralVariant=Passthrough  ExternalSaturationOutDataTypeStr=Inherit: Same as second input
  ParkClarke : Subsystem
  Sum : Sum  Inputs=|+-
  Sum1 : Sum  Inputs=-+|
  v_cmd : Outport
  wires:
  i_d command/1 -> Sum/1
  i_q command/1 -> Sum1/2
  Sum/1 -> PID Controller/1
  Sum1/1 -> PID Controller1/1
  Phase A angle/1 -> InvParkClarke/3(theta), ParkClarke/2(theta)
  InvParkClarke/1(abc) -> v_cmd/1
  Three-phase current/1 -> ParkClarke/1(abc)
  ParkClarke/1(Id) -> Sum/2  "Id_meas"
  ParkClarke/2(Iq) -> Sum1/1  "Iq_meas"
  PID Controller/1 -> Decoupling/1(Id_coupled)
  PID Controller1/1 -> Decoupling/2(Iq_coupled)
  Decoupling/1(Id_uncoupled) -> InvParkClarke/1(Id)
  Electrical speed/1 -> Decoupling/3(Electrical speed)
  Decoupling/2(Iq_uncoupled) -> InvParkClarke/2(Iq)

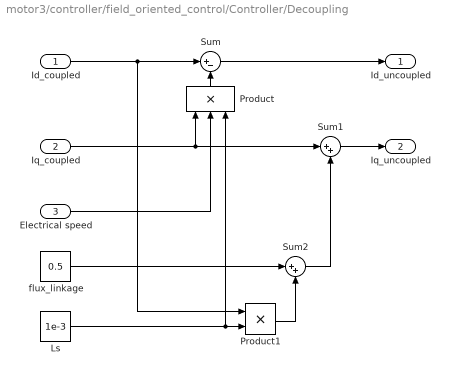
== system motor3/controller/field_oriented_control/Controller/Decoupling ==
  Id_coupled : Inport
  Iq_coupled : Inport  Port=2
  Electrical speed : Inport  Port=3
  Ls : Constant  Value=1e-3
  Product : Product  Inputs=3
  Product1 : Product
  Sum : Sum  Inputs=|+-
  Sum1 : Sum  Inputs=|++
  Sum2 : Sum  Inputs=|++
  flux_linkage : Constant  Value=0.5
  Id_uncoupled : Outport
  Iq_uncoupled : Outport  Port=2
  wires:
  Id_coupled/1 -> Product1/1, Sum/1
  Electrical speed/1 -> Product/2
  Ls/1 -> Product/3, Product1/2
  Product/1 -> Sum/2
  Iq_coupled/1 -> Product/1, Sum1/1
  Product1/1 -> Sum2/2
  flux_linkage/1 -> Sum2/1
  Sum2/1 -> Sum1/2
  Sum/1 -> Id_uncoupled/1
  Sum1/1 -> Iq_uncoupled/1

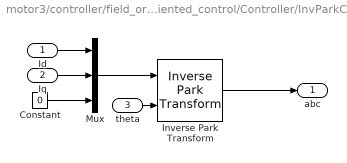
== system motor3/controller/field_oriented_control/Controller/InvParkClarke ==
  Id : Inport
  Iq : Inport  Port=2
  theta : Inport  Port=3
  Constant : Constant  Value=0
  Inverse Park Transform : eeTransforms/Inverse Park Transform  AxisAlignment=Q-axis  PowerInvariant=off
  Mux : Mux  Inputs=3
  abc : Outport
  wires:
  Iq/1 -> Mux/2
  Constant/1 -> Mux/3
  Mux/1 -> Inverse Park Transform/1
  theta/1 -> Inverse Park Transform/2
  Inverse Park Transform/1 -> abc/1
  Id/1 -> Mux/1

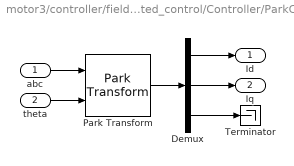
== system motor3/controller/field_oriented_control/Controller/ParkClarke ==
  abc : Inport
  theta : Inport  Port=2
  Demux : Demux  Outputs=3
  Park Transform : eeTransforms/Park Transform  AxisAlignment=Q-axis  PowerInvariant=off
  Terminator : Terminator
  Id : Outport
  Iq : Outport  Port=2
  wires:
  Demux/1 -> Id/1
  Park Transform/1 -> Demux/1
  Demux/2 -> Iq/1
  theta/1 -> Park Transform/2
  Demux/3 -> Terminator/1
  abc/1 -> Park Transform/1
